simulink model "LQR_Gain_Scheduled_step"  (R2019a)
settings: Solver=VariableStepAuto  StartTime=0.0  StopTime=2.5  FixedStep=-1  RelTol=1e-3
values from neighbouring files (symbols this model uses):
  Cf = 30989.0    [LQR.sldd]    (also in LQR_Gain_Scheduled_Setup.m = 30989)
  Cr = 50154.0    [LQR.sldd]    (also in LQR_Gain_Scheduled_Setup.m = 50154)
  Iz = 111.8    [LQR.sldd]    (also in LQR_Gain_Scheduled_Setup.m)
  K1 = 2.2904418292062911 1.8847463893542393 1.3242417081766078 0.62878568102574306 -0.1585896057605396    [LQR.sldd]
  K2 = 6.3913014514393458 6.6677491042301451 6.8847629785684639 7.1165672340645614 7.3671824821430132    [LQR.sldd]
  K3 = -83.66600265340719 -83.66600265340729 -83.66600265340999 -83.666002653406792 -83.666002653407688    [LQR.sldd]
  lf = 0.783    [LQR.sldd]    (also in LQR_Gain_Scheduled_Setup.m)
  lr = 0.752    [LQR.sldd]    (also in LQR_Gain_Scheduled_Setup.m)
  m = 245.0    [LQR.sldd]    (also in LQR_Gain_Scheduled_Setup.m = 245)
settings Model: DataDictionary=LQR.sldd  EnableAccessToBaseWorkspace=off  Creator=Johan PC  LastModifiedBy=Johan PC
settings DataIOCC: ReturnWorkspaceOutputs=off
settings DebuggingCC: ArithmeticOperatorsInVariantConditions=warning

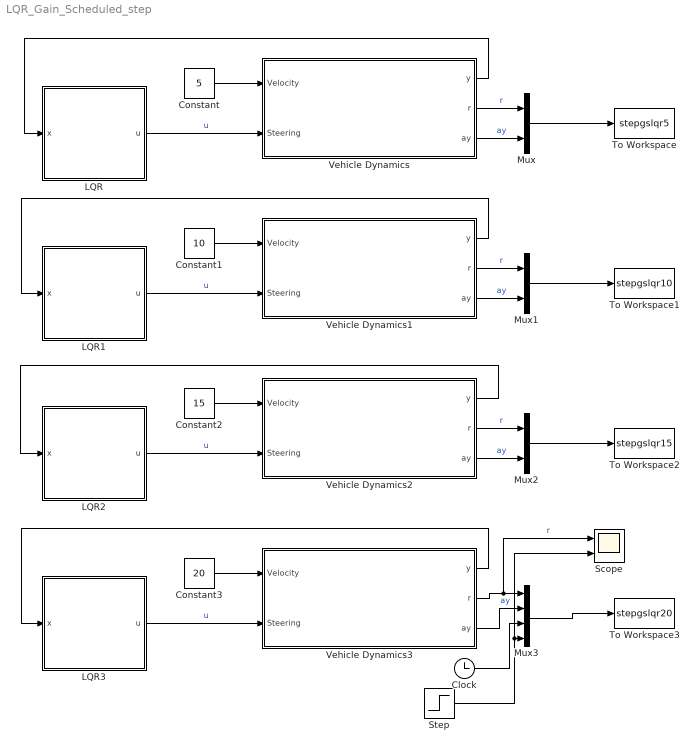
== system LQR_Gain_Scheduled_step ==
  Clock : Clock
      settings: Decimation=3
  Constant : Constant  Value=5
  Constant1 : Constant  Value=10
  Constant2 : Constant  Value=15
  Constant3 : Constant  Value=20
  LQR : Subsystem
  LQR1 : Subsystem
  LQR2 : Subsystem
  LQR3 : Subsystem
  Mux : Mux  Inputs=2
  Mux1 : Mux  Inputs=2
  Mux2 : Mux  Inputs=2
  Mux3 : Mux
  Scope : Scope  NumInputPorts=2
  Step : Step  Time=0.5  SampleTime=0
  To Workspace : ToWorkspace  VariableName=stepgslqr5  SampleTime=0.01
      settings: Save2DSignal=2-D array (concatenate along first dimension)
  To Workspace1 : ToWorkspace  VariableName=stepgslqr10  SampleTime=0.01
      settings: Save2DSignal=2-D array (concatenate along first dimension)
  To Workspace2 : ToWorkspace  VariableName=stepgslqr15  SampleTime=0.01
  To Workspace3 : ToWorkspace  VariableName=stepgslqr20  SampleTime=0.01
      settings: Save2DSignal=2-D array (concatenate along first dimension)
  Vehicle Dynamics : Subsystem
  Vehicle Dynamics1 : Subsystem
  Vehicle Dynamics2 : Subsystem
  Vehicle Dynamics3 : Subsystem
  wires:
  Vehicle Dynamics/1("y ") -> LQR/1(x)
  LQR/1(u) -> Vehicle Dynamics/2(Steering)  "u"
  Vehicle Dynamics/3(ay) -> Mux/2  "ay"
  Vehicle Dynamics/2("r ") -> Mux/1  "r"
  Constant/1 -> Vehicle Dynamics/1(Velocity)
  Mux/1 -> To Workspace/1
  Constant1/1 -> Vehicle Dynamics1/1(Velocity)
  LQR1/1(u) -> Vehicle Dynamics1/2(Steering)  "u"
  Mux1/1 -> To Workspace1/1
  Vehicle Dynamics1/1("y ") -> LQR1/1(x)
  Vehicle Dynamics1/2("r ") -> Mux1/1  "r"
  Vehicle Dynamics1/3(ay) -> Mux1/2  "ay"
  Constant2/1 -> Vehicle Dynamics2/1(Velocity)
  LQR2/1(u) -> Vehicle Dynamics2/2(Steering)  "u"
  Mux2/1 -> To Workspace2/1
  Vehicle Dynamics2/1("y ") -> LQR2/1(x)
  Vehicle Dynamics2/2("r ") -> Mux2/1  "r"
  Vehicle Dynamics2/3(ay) -> Mux2/2  "ay"
  Constant3/1 -> Vehicle Dynamics3/1(Velocity)
  LQR3/1(u) -> Vehicle Dynamics3/2(Steering)  "u"
  Mux3/1 -> To Workspace3/1
  Vehicle Dynamics3/1("y ") -> LQR3/1(x)
  Vehicle Dynamics3/2("r ") -> Scope/1, Mux3/1  "r"
  Vehicle Dynamics3/3(ay) -> Mux3/2  "ay"
  Clock/1 -> Mux3/3
  Step/1 -> Scope/2, Mux3/4

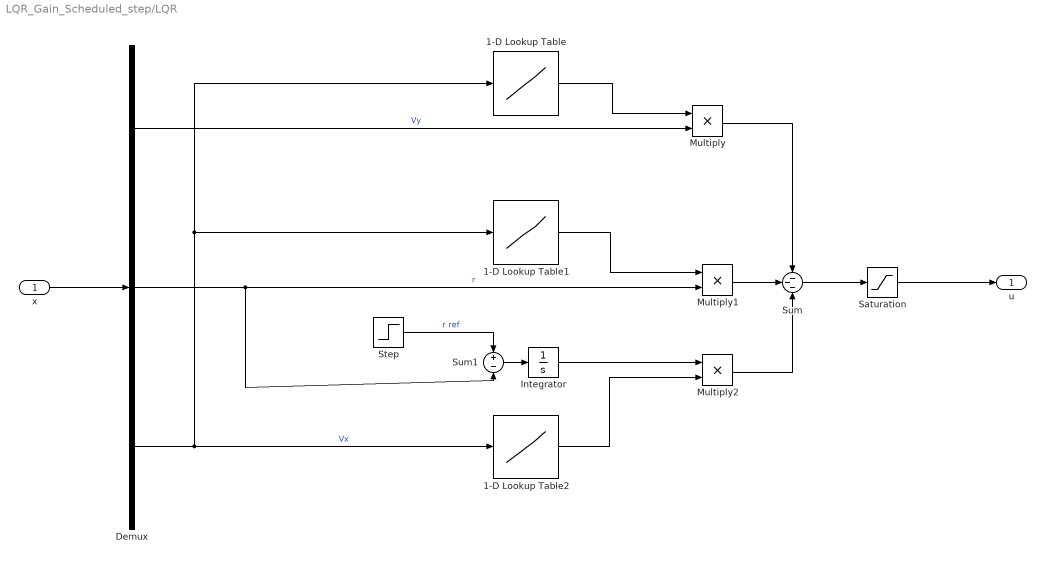
== system LQR_Gain_Scheduled_step/LQR ==
  x : Inport
  1-D Lookup Table : Lookup_n-D  NumberOfTableDimensions=1  BreakpointsSpecification=Even spacing  BreakpointsForDimension1=[-5:5]  BreakpointsForDimension1FirstPoint=5  BreakpointsForDimension1Spacing=5  Table=K1  InterpMethod=Flat  InternalRulePriority=Speed  RndMeth=Simplest  InputSameDT=on
  1-D Lookup Table1 : Lookup_n-D  NumberOfTableDimensions=1  BreakpointsSpecification=Even spacing  BreakpointsForDimension1=[-5:5]  BreakpointsForDimension1FirstPoint=5  BreakpointsForDimension1Spacing=5  Table=K2  InterpMethod=Flat  InternalRulePriority=Speed  RndMeth=Simplest  InputSameDT=on
  1-D Lookup Table2 : Lookup_n-D  NumberOfTableDimensions=1  BreakpointsSpecification=Even spacing  BreakpointsForDimension1=[-5:5]  BreakpointsForDimension1FirstPoint=5  BreakpointsForDimension1Spacing=5  Table=K3  InternalRulePriority=Speed  RndMeth=Simplest  InputSameDT=on
  Demux : Demux  Outputs=3
  Integrator : Integrator
  Multiply : Product
  Multiply1 : Product
  Multiply2 : Product
  Saturation : Saturate  UpperLimit=0.45  LowerLimit=-0.45
  Step : Step  Time=0.5  SampleTime=0
  Sum : Sum  Inputs=---
  Sum1 : Sum  Inputs=+-
  u : Outport
  wires:
  Integrator/1 -> Multiply2/1
  Multiply2/1 -> Sum/3
  x/1 -> Demux/1
  Demux/2 -> Multiply1/2, Sum1/2  "r"
  Multiply/1 -> Sum/1
  Multiply1/1 -> Sum/2
  Sum/1 -> Saturation/1
  Sum1/1 -> Integrator/1
  Step/1 -> Sum1/1  "r ref"
  Saturation/1 -> u/1
  1-D Lookup Table/1 -> Multiply/1
  Demux/1 -> Multiply/2  "Vy"
  Demux/3 -> 1-D Lookup Table/1, 1-D Lookup Table1/1, 1-D Lookup Table2/1  "Vx"
  1-D Lookup Table1/1 -> Multiply1/1
  1-D Lookup Table2/1 -> Multiply2/2

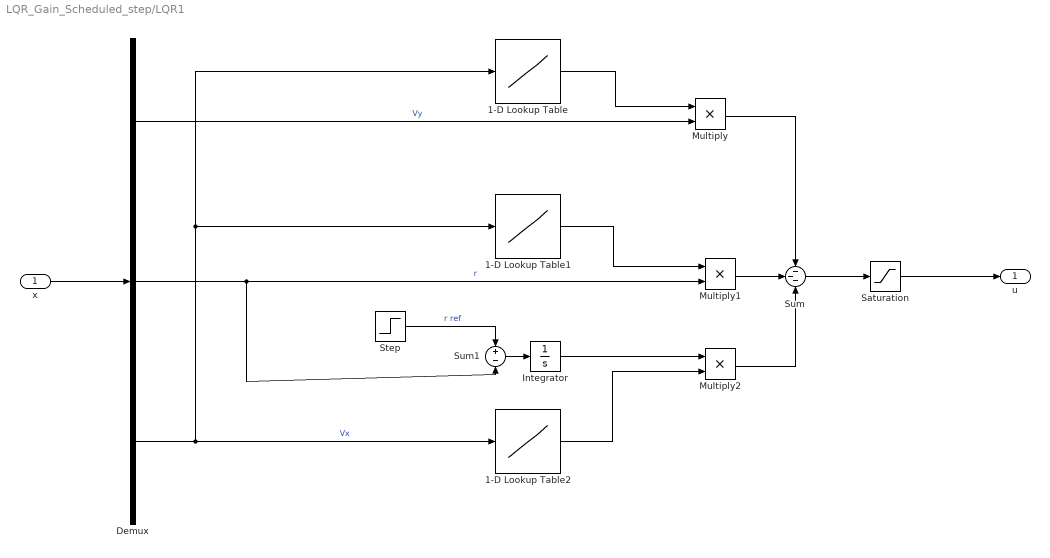
== system LQR_Gain_Scheduled_step/LQR1 ==
  x : Inport
  1-D Lookup Table : Lookup_n-D  NumberOfTableDimensions=1  BreakpointsSpecification=Even spacing  BreakpointsForDimension1=[-5:5]  BreakpointsForDimension1FirstPoint=5  BreakpointsForDimension1Spacing=5  Table=K1  InternalRulePriority=Speed  RndMeth=Simplest  InputSameDT=on
  1-D Lookup Table1 : Lookup_n-D  NumberOfTableDimensions=1  BreakpointsSpecification=Even spacing  BreakpointsForDimension1=[-5:5]  BreakpointsForDimension1FirstPoint=5  BreakpointsForDimension1Spacing=5  Table=K2  InternalRulePriority=Speed  RndMeth=Simplest  InputSameDT=on
  1-D Lookup Table2 : Lookup_n-D  NumberOfTableDimensions=1  BreakpointsSpecification=Even spacing  BreakpointsForDimension1=[-5:5]  BreakpointsForDimension1FirstPoint=5  BreakpointsForDimension1Spacing=5  Table=K3  InternalRulePriority=Speed  RndMeth=Simplest  InputSameDT=on
  Demux : Demux  Outputs=3
  Integrator : Integrator
  Multiply : Product
  Multiply1 : Product
  Multiply2 : Product
  Saturation : Saturate  UpperLimit=0.45  LowerLimit=-0.45
  Step : Step  Time=0.5  SampleTime=0
  Sum : Sum  Inputs=---
  Sum1 : Sum  Inputs=+-
  u : Outport
  wires:
  Integrator/1 -> Multiply2/1
  Multiply2/1 -> Sum/3
  x/1 -> Demux/1
  Demux/2 -> Multiply1/2, Sum1/2  "r"
  Multiply/1 -> Sum/1
  Multiply1/1 -> Sum/2
  Sum/1 -> Saturation/1
  Sum1/1 -> Integrator/1
  Step/1 -> Sum1/1  "r ref"
  Saturation/1 -> u/1
  1-D Lookup Table/1 -> Multiply/1
  Demux/1 -> Multiply/2  "Vy"
  Demux/3 -> 1-D Lookup Table/1, 1-D Lookup Table1/1, 1-D Lookup Table2/1  "Vx"
  1-D Lookup Table1/1 -> Multiply1/1
  1-D Lookup Table2/1 -> Multiply2/2

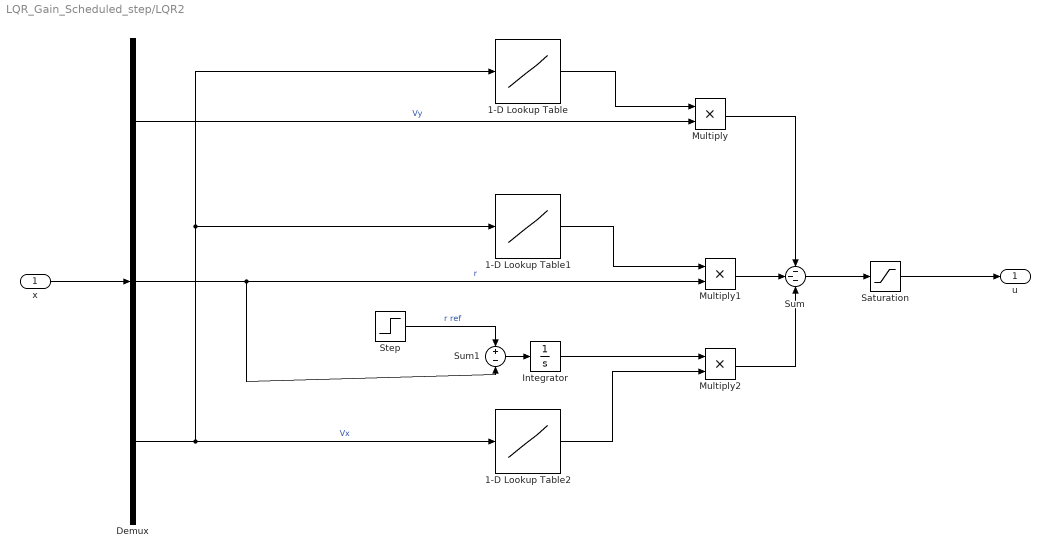
== system LQR_Gain_Scheduled_step/LQR2 ==
  x : Inport
  1-D Lookup Table : Lookup_n-D  NumberOfTableDimensions=1  BreakpointsSpecification=Even spacing  BreakpointsForDimension1=[-5:5]  BreakpointsForDimension1FirstPoint=5  BreakpointsForDimension1Spacing=5  Table=K1  InternalRulePriority=Speed  RndMeth=Simplest  InputSameDT=on
  1-D Lookup Table1 : Lookup_n-D  NumberOfTableDimensions=1  BreakpointsSpecification=Even spacing  BreakpointsForDimension1=[-5:5]  BreakpointsForDimension1FirstPoint=5  BreakpointsForDimension1Spacing=5  Table=K2  InternalRulePriority=Speed  RndMeth=Simplest  InputSameDT=on
  1-D Lookup Table2 : Lookup_n-D  NumberOfTableDimensions=1  BreakpointsSpecification=Even spacing  BreakpointsForDimension1=[-5:5]  BreakpointsForDimension1FirstPoint=5  BreakpointsForDimension1Spacing=5  Table=K3  InternalRulePriority=Speed  RndMeth=Simplest  InputSameDT=on
  Demux : Demux  Outputs=3
  Integrator : Integrator
  Multiply : Product
  Multiply1 : Product
  Multiply2 : Product
  Saturation : Saturate  UpperLimit=0.45  LowerLimit=-0.45
  Step : Step  Time=0.5  SampleTime=0
  Sum : Sum  Inputs=---
  Sum1 : Sum  Inputs=+-
  u : Outport
  wires:
  Integrator/1 -> Multiply2/1
  Multiply2/1 -> Sum/3
  x/1 -> Demux/1
  Demux/2 -> Multiply1/2, Sum1/2  "r"
  Multiply/1 -> Sum/1
  Multiply1/1 -> Sum/2
  Sum/1 -> Saturation/1
  Sum1/1 -> Integrator/1
  Step/1 -> Sum1/1  "r ref"
  Saturation/1 -> u/1
  1-D Lookup Table/1 -> Multiply/1
  Demux/1 -> Multiply/2  "Vy"
  Demux/3 -> 1-D Lookup Table/1, 1-D Lookup Table1/1, 1-D Lookup Table2/1  "Vx"
  1-D Lookup Table1/1 -> Multiply1/1
  1-D Lookup Table2/1 -> Multiply2/2

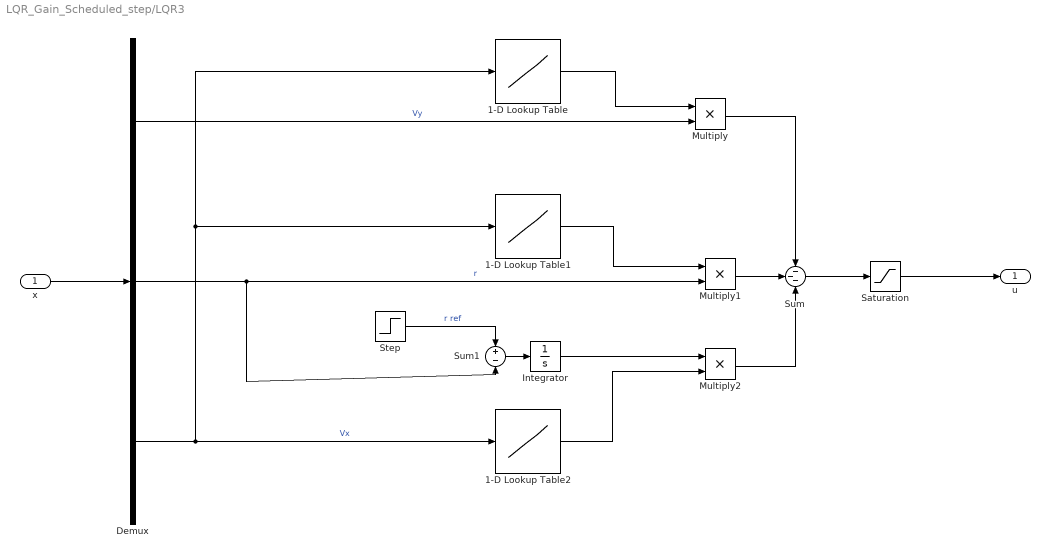
== system LQR_Gain_Scheduled_step/LQR3 ==
  x : Inport
  1-D Lookup Table : Lookup_n-D  NumberOfTableDimensions=1  BreakpointsSpecification=Even spacing  BreakpointsForDimension1=[-5:5]  BreakpointsForDimension1FirstPoint=5  BreakpointsForDimension1Spacing=5  Table=K1  InternalRulePriority=Speed  RndMeth=Simplest  InputSameDT=on
  1-D Lookup Table1 : Lookup_n-D  NumberOfTableDimensions=1  BreakpointsSpecification=Even spacing  BreakpointsForDimension1=[-5:5]  BreakpointsForDimension1FirstPoint=5  BreakpointsForDimension1Spacing=5  Table=K2  InternalRulePriority=Speed  RndMeth=Simplest  InputSameDT=on
  1-D Lookup Table2 : Lookup_n-D  NumberOfTableDimensions=1  BreakpointsSpecification=Even spacing  BreakpointsForDimension1=[-5:5]  BreakpointsForDimension1FirstPoint=5  BreakpointsForDimension1Spacing=5  Table=K3  InternalRulePriority=Speed  RndMeth=Simplest  InputSameDT=on
  Demux : Demux  Outputs=3
  Integrator : Integrator
  Multiply : Product
  Multiply1 : Product
  Multiply2 : Product
  Saturation : Saturate  UpperLimit=0.45  LowerLimit=-0.45
  Step : Step  Time=0.5  SampleTime=0
  Sum : Sum  Inputs=---
  Sum1 : Sum  Inputs=+-
  u : Outport
  wires:
  Integrator/1 -> Multiply2/1
  Multiply2/1 -> Sum/3
  x/1 -> Demux/1
  Demux/2 -> Multiply1/2, Sum1/2  "r"
  Multiply/1 -> Sum/1
  Multiply1/1 -> Sum/2
  Sum/1 -> Saturation/1
  Sum1/1 -> Integrator/1
  Step/1 -> Sum1/1  "r ref"
  Saturation/1 -> u/1
  1-D Lookup Table/1 -> Multiply/1
  Demux/1 -> Multiply/2  "Vy"
  Demux/3 -> 1-D Lookup Table/1, 1-D Lookup Table1/1, 1-D Lookup Table2/1  "Vx"
  1-D Lookup Table1/1 -> Multiply1/1
  1-D Lookup Table2/1 -> Multiply2/2

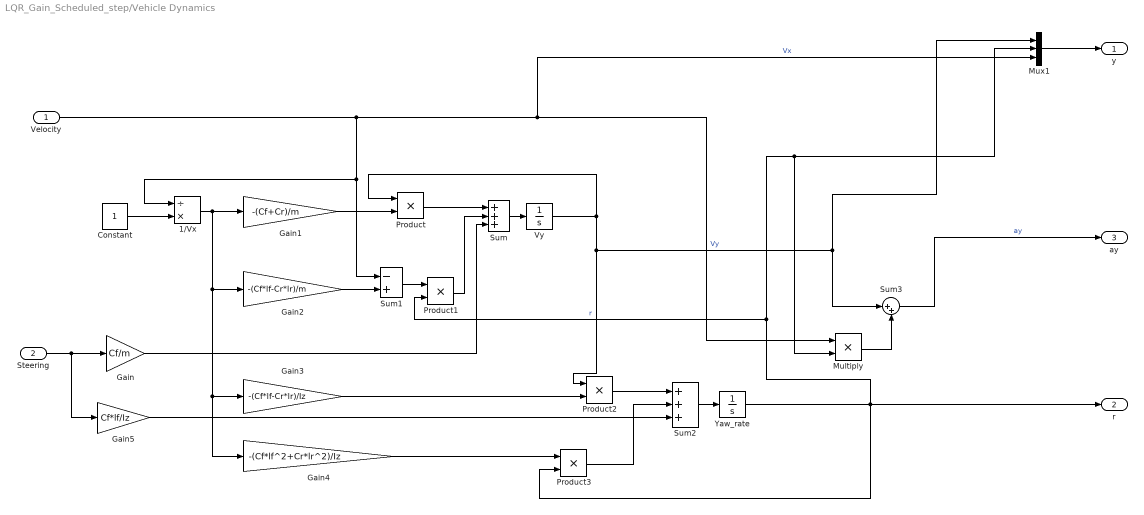
== system LQR_Gain_Scheduled_step/Vehicle Dynamics ==
  Velocity : Inport
  Steering : Inport  Port=2
  1/Vx : Product  Inputs=/*
  Constant : Constant
  Gain : Gain  Gain=Cf/m
  Gain1 : Gain  Gain=-(Cf+Cr)/m
  Gain2 : Gain  Gain=-(Cf*lf-Cr*lr)/m
  Gain3 : Gain  Gain=-(Cf*lf-Cr*lr)/Iz
  Gain4 : Gain  Gain=-(Cf*lf^2+Cr*lr^2)/Iz
  Gain5 : Gain  Gain=Cf*lf/Iz
  Multiply : Product
  Mux1 : Mux  Inputs=3
  Product{,1..3} (4 alike) : Product
  Sum : Sum  Inputs=+++
  Sum1 : Sum  Inputs=-+
  Sum2 : Sum  Inputs=+++
  Sum3 : Sum  Inputs=|++
  Vy : Integrator
  "Yaw_rate " : Integrator
  "y " : Outport
  "r " : Outport  Port=2
  ay : Outport  Port=3
  wires:
  Sum2/1 -> "Yaw_rate "/1
  Gain2/1 -> Sum1/2
  Gain4/1 -> Product3/1
  Constant/1 -> 1/Vx/2
  Gain3/1 -> Product2/2
  1/Vx/1 -> Gain4/1, Gain3/1, Gain2/1, Gain1/1
  Product2/1 -> Sum2/1
  Product3/1 -> Sum2/2
  Gain5/1 -> Sum2/3
  Sum1/1 -> Product1/1
  "Yaw_rate "/1 -> Multiply/2, Mux1/2, Product1/2, "r "/1, Product3/2  "r"
  Gain/1 -> Sum/3
  Steering/1 -> Gain/1, Gain5/1
  Gain1/1 -> Product/2
  Product/1 -> Sum/1
  Vy/1 -> Mux1/1, Sum3/1, Product2/1, Product/1  "Vy"
  Sum/1 -> Vy/1
  Velocity/1 -> Mux1/3, Multiply/1, 1/Vx/1, Sum1/1  "Vx"
  Product1/1 -> Sum/2
  Multiply/1 -> Sum3/2
  Sum3/1 -> ay/1  "ay"
  Mux1/1 -> "y "/1

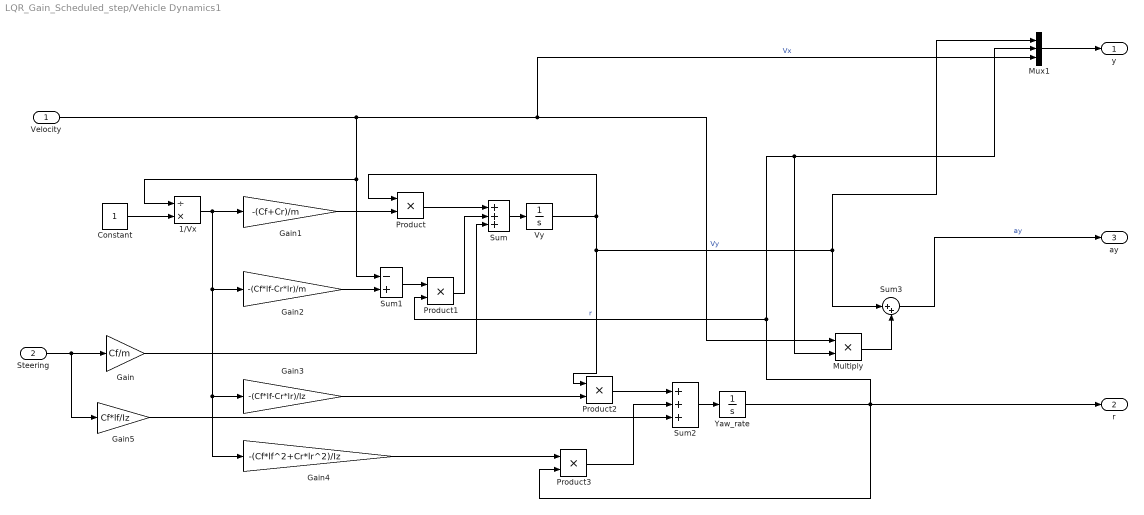
== system LQR_Gain_Scheduled_step/Vehicle Dynamics1 ==
  Velocity : Inport
  Steering : Inport  Port=2
  1/Vx : Product  Inputs=/*
  Constant : Constant
  Gain : Gain  Gain=Cf/m
  Gain1 : Gain  Gain=-(Cf+Cr)/m
  Gain2 : Gain  Gain=-(Cf*lf-Cr*lr)/m
  Gain3 : Gain  Gain=-(Cf*lf-Cr*lr)/Iz
  Gain4 : Gain  Gain=-(Cf*lf^2+Cr*lr^2)/Iz
  Gain5 : Gain  Gain=Cf*lf/Iz
  Multiply : Product
  Mux1 : Mux  Inputs=3
  Product{,1..3} (4 alike) : Product
  Sum : Sum  Inputs=+++
  Sum1 : Sum  Inputs=-+
  Sum2 : Sum  Inputs=+++
  Sum3 : Sum  Inputs=|++
  Vy : Integrator
  "Yaw_rate " : Integrator
  "y " : Outport
  "r " : Outport  Port=2
  ay : Outport  Port=3
  wires:
  Mux1/1 -> "y "/1
  Sum3/1 -> ay/1  "ay"
  Multiply/1 -> Sum3/2
  Product1/1 -> Sum/2
  Velocity/1 -> Sum1/1, 1/Vx/1, Multiply/1, Mux1/3  "Vx"
  Sum/1 -> Vy/1
  Vy/1 -> Product/1, Product2/1, Sum3/1, Mux1/1  "Vy"
  Product/1 -> Sum/1
  Gain1/1 -> Product/2
  Steering/1 -> Gain5/1, Gain/1
  Gain/1 -> Sum/3
  "Yaw_rate "/1 -> Product3/2, "r "/1, Product1/2, Mux1/2, Multiply/2  "r"
  Sum1/1 -> Product1/1
  Gain5/1 -> Sum2/3
  Product3/1 -> Sum2/2
  Product2/1 -> Sum2/1
  1/Vx/1 -> Gain1/1, Gain2/1, Gain3/1, Gain4/1
  Gain3/1 -> Product2/2
  Constant/1 -> 1/Vx/2
  Gain4/1 -> Product3/1
  Gain2/1 -> Sum1/2
  Sum2/1 -> "Yaw_rate "/1

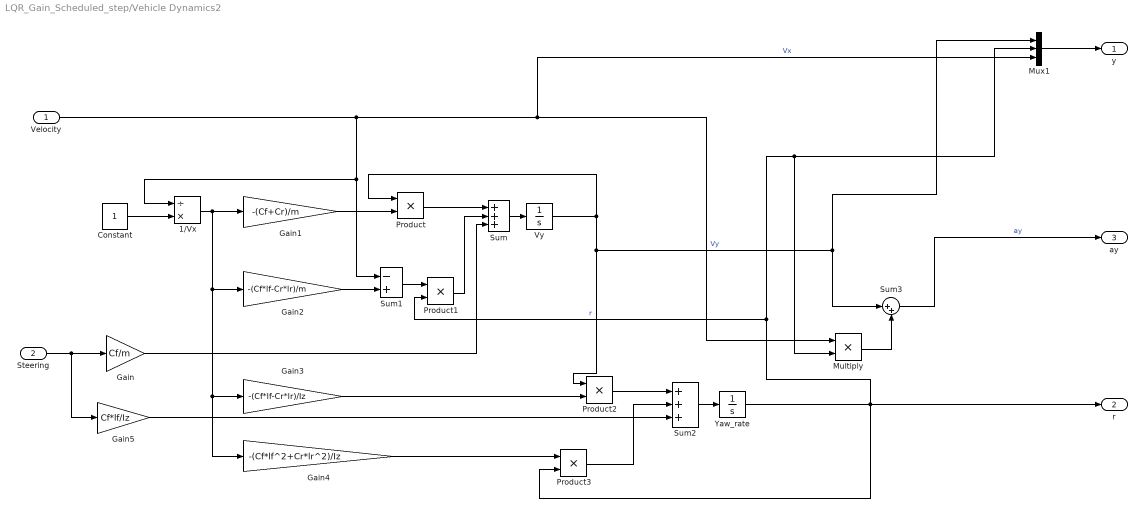
== system LQR_Gain_Scheduled_step/Vehicle Dynamics2 ==
  Velocity : Inport
  Steering : Inport  Port=2
  1/Vx : Product  Inputs=/*
  Constant : Constant
  Gain : Gain  Gain=Cf/m
  Gain1 : Gain  Gain=-(Cf+Cr)/m
  Gain2 : Gain  Gain=-(Cf*lf-Cr*lr)/m
  Gain3 : Gain  Gain=-(Cf*lf-Cr*lr)/Iz
  Gain4 : Gain  Gain=-(Cf*lf^2+Cr*lr^2)/Iz
  Gain5 : Gain  Gain=Cf*lf/Iz
  Multiply : Product
  Mux1 : Mux  Inputs=3
  Product{,1..3} (4 alike) : Product
  Sum : Sum  Inputs=+++
  Sum1 : Sum  Inputs=-+
  Sum2 : Sum  Inputs=+++
  Sum3 : Sum  Inputs=|++
  Vy : Integrator
  "Yaw_rate " : Integrator
  "y " : Outport
  "r " : Outport  Port=2
  ay : Outport  Port=3
  wires:
  Sum2/1 -> "Yaw_rate "/1
  Gain2/1 -> Sum1/2
  Gain4/1 -> Product3/1
  Constant/1 -> 1/Vx/2
  Gain3/1 -> Product2/2
  1/Vx/1 -> Gain4/1, Gain3/1, Gain2/1, Gain1/1
  Product2/1 -> Sum2/1
  Product3/1 -> Sum2/2
  Gain5/1 -> Sum2/3
  Sum1/1 -> Product1/1
  "Yaw_rate "/1 -> Multiply/2, Mux1/2, Product1/2, "r "/1, Product3/2  "r"
  Gain/1 -> Sum/3
  Steering/1 -> Gain/1, Gain5/1
  Gain1/1 -> Product/2
  Product/1 -> Sum/1
  Vy/1 -> Mux1/1, Sum3/1, Product2/1, Product/1  "Vy"
  Sum/1 -> Vy/1
  Velocity/1 -> Mux1/3, Multiply/1, 1/Vx/1, Sum1/1  "Vx"
  Product1/1 -> Sum/2
  Multiply/1 -> Sum3/2
  Sum3/1 -> ay/1  "ay"
  Mux1/1 -> "y "/1

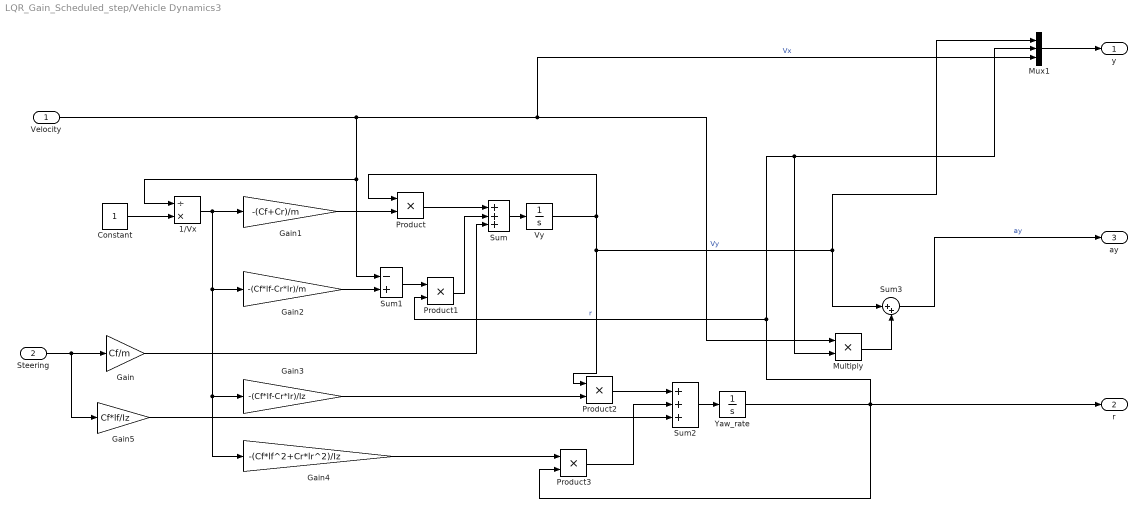
== system LQR_Gain_Scheduled_step/Vehicle Dynamics3 ==
  Velocity : Inport
  Steering : Inport  Port=2
  1/Vx : Product  Inputs=/*
  Constant : Constant
  Gain : Gain  Gain=Cf/m
  Gain1 : Gain  Gain=-(Cf+Cr)/m
  Gain2 : Gain  Gain=-(Cf*lf-Cr*lr)/m
  Gain3 : Gain  Gain=-(Cf*lf-Cr*lr)/Iz
  Gain4 : Gain  Gain=-(Cf*lf^2+Cr*lr^2)/Iz
  Gain5 : Gain  Gain=Cf*lf/Iz
  Multiply : Product
  Mux1 : Mux  Inputs=3
  Product{,1..3} (4 alike) : Product
  Sum : Sum  Inputs=+++
  Sum1 : Sum  Inputs=-+
  Sum2 : Sum  Inputs=+++
  Sum3 : Sum  Inputs=|++
  Vy : Integrator
  "Yaw_rate " : Integrator
  "y " : Outport
  "r " : Outport  Port=2
  ay : Outport  Port=3
  wires:
  Mux1/1 -> "y "/1
  Sum3/1 -> ay/1  "ay"
  Multiply/1 -> Sum3/2
  Product1/1 -> Sum/2
  Velocity/1 -> Sum1/1, 1/Vx/1, Multiply/1, Mux1/3  "Vx"
  Sum/1 -> Vy/1
  Vy/1 -> Product/1, Product2/1, Sum3/1, Mux1/1  "Vy"
  Product/1 -> Sum/1
  Gain1/1 -> Product/2
  Steering/1 -> Gain5/1, Gain/1
  Gain/1 -> Sum/3
  "Yaw_rate "/1 -> Product3/2, "r "/1, Product1/2, Mux1/2, Multiply/2  "r"
  Sum1/1 -> Product1/1
  Gain5/1 -> Sum2/3
  Product3/1 -> Sum2/2
  Product2/1 -> Sum2/1
  1/Vx/1 -> Gain1/1, Gain2/1, Gain3/1, Gain4/1
  Gain3/1 -> Product2/2
  Constant/1 -> 1/Vx/2
  Gain4/1 -> Product3/1
  Gain2/1 -> Sum1/2
  Sum2/1 -> "Yaw_rate "/1
